simulink model "example3"  (Simulink 7.5)
settings: Solver=ode45  StartTime=0.0  StopTime=0.5  RelTol=1e-3
undefined symbols (not defined in the file or in its folder): deriv_fcn, x0
settings Model: Creator=rhanz  LastModifiedBy=rhanz

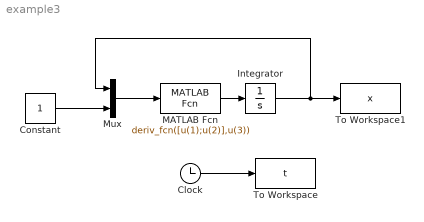
== system example3 ==
  Clock : Clock
      settings: Decimation=10
  Constant : Constant  OutDataType=fixdt(1, 16)  OutScaling=2^0
  Integrator : Integrator  InitialCondition=x0
  MATLAB Fcn : MATLABFcn  MATLABFcn=deriv_fcn([u(1);u(2)],u(3))
  Mux : Mux  Inputs=2
  To Workspace : ToWorkspace  VariableName=t  SampleTime=-1  SaveFormat=Array
  To Workspace1 : ToWorkspace  VariableName=x  SampleTime=-1  SaveFormat=Array
  wires:
  MATLAB Fcn/1 -> Integrator/1
  Mux/1 -> MATLAB Fcn/1
  Constant/1 -> Mux/2
  Integrator/1 -> Mux/1, To Workspace1/1
  Clock/1 -> To Workspace/1
